simulink model "SHA256_simulink"  (R2015a)
settings: Solver=ode3  StartTime=0.0  StopTime=0  RelTol=1e-3
libraries: simulink x34, hdlsllib x24
settings Model: Creator=Hp  LastModifiedBy=Hp

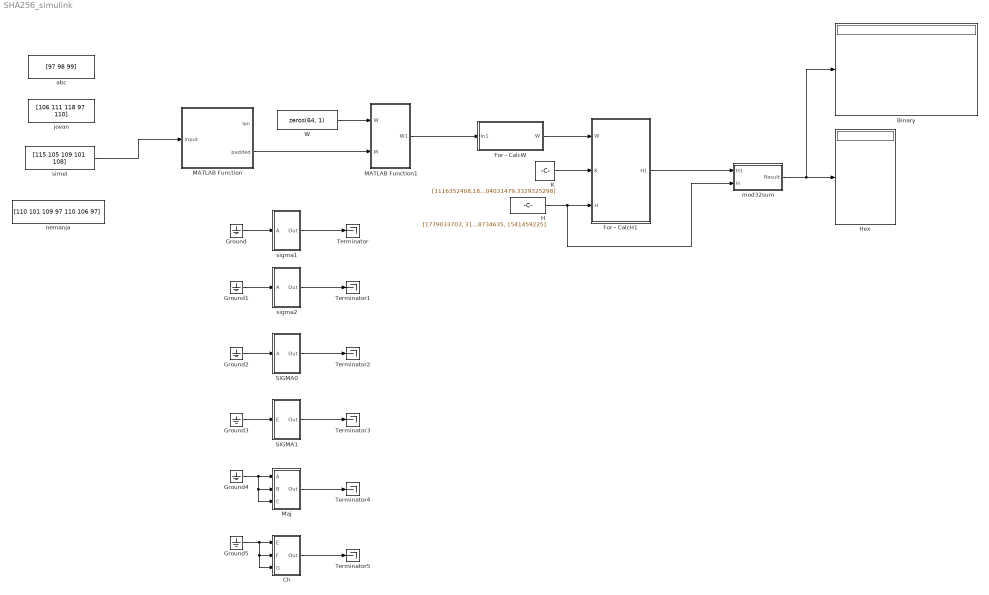
== system SHA256_simulink ==
  Binary : Display
      settings: Format=binary (Stored Integer)
  Ch : Subsystem
  For - CalcH1 : Subsystem  TreatAsAtomicUnit=on
  For - CalcW : Subsystem  TreatAsAtomicUnit=on
  Ground{,1..5} (6 alike) : Ground
  H : Constant  Value=[1779033703, 3144134277, 1013904242, 2773480762, 1359893119, 2600822924, 528734635, 1541459225]  OutDataTypeStr=uint32
  Hex : Display
      settings: Format=hex (Stored Integer)
  K : Constant  Value=[1116352408,1899447441,3049323471,3921009573,961987163,1508970993,2453635748,2870763221,3624381080,310598401,607225278,1426881987,1925078388,2162078206,2614888103,3248222580,3835390401,4022224774,264347078,604807628,770255983,1249150122,1555081692,1996064986,2554220882,2821834349,2952996808,3210313671,3336571891,3584528711,113926993,338241895,666307205,773529912,1294757372,1396182291,1695183700,1986661051,2177026350,2456956037,2730485921,2820302411,3259730800,3345764771,3516065817,3600352804,4094571909,275423344,430227734,506948616,659060556,883997877,958139571,1322822218,1537002063,1747873779,1955562222,2024104815,2227730452,2361852424,2428436474,2756734187,3204031479,3329325298]  OutDataTypeStr=uint32
  MATLAB Function : MATLAB Function  TreatAsAtomicUnit=on
  MATLAB Function1 : MATLAB Function  TreatAsAtomicUnit=on
  Maj : Subsystem
  SIGMA0 : Subsystem
  SIGMA1 : Subsystem
  Terminator{,1..5} (6 alike) : Terminator
  W : Constant  Value=zeros(64, 1)  VectorParams1D=off  OutDataTypeStr=uint32
  abc : Constant  Value=[97 98 99]
  jovan : Constant  Value=[106 111 118 97 110]
  mod32sum : Subsystem
  nemanja : Constant  Value=[110 101 109 97 110 106 97]
  "sigma1 " : Subsystem
  sigma2 : Subsystem
  "simel " : Constant  Value=[115 105 109 101 108]
  wires:
  W/1 -> MATLAB Function1/1(W)
  MATLAB Function/2(padded) -> MATLAB Function1/2(M)
  For - CalcW/1(W) -> For - CalcH1/1(W)
  K/1 -> For - CalcH1/2(K)
  For - CalcH1/1(H1) -> mod32sum/1(H1)
  mod32sum/1(Result) -> Binary/1, Hex/1
  H/1 -> mod32sum/2(H), For - CalcH1/3(H)
  Ground/1 -> "sigma1 "/1(A)
  Ground1/1 -> sigma2/1(A)
  Ground2/1 -> SIGMA0/1(A)
  Ground3/1 -> SIGMA1/1(E)
  Ground4/1 -> Maj/3(C), Maj/2(B), Maj/1(A)
  Ground5/1 -> Ch/3(G), Ch/2(F), Ch/1(E)
  "sigma1 "/1(Out) -> Terminator/1
  sigma2/1(Out) -> Terminator1/1
  SIGMA0/1(Out) -> Terminator2/1
  SIGMA1/1(Out) -> Terminator3/1
  Maj/1(Out) -> Terminator4/1
  Ch/1(Out) -> Terminator5/1
  "simel "/1 -> MATLAB Function/1(input)
  MATLAB Function1/1(W1) -> For - CalcW/1(In1)

== system SHA256_simulink/Ch ==
  E : Inport  OutDataTypeStr=uint32
  F : Inport  Port=2  OutDataTypeStr=uint32
  G : Inport  Port=3  OutDataTypeStr=uint32
  Bitwise Operator1 : simulink/Logic and Bit Operations/Bitwise Operator  logicop=AND  UseBitMask=off  NumInputPorts=2  BitMask=bin2dec('11011001')  BitMaskRealWorld=Stored Integer
  Bitwise Operator2 : simulink/Logic and Bit Operations/Bitwise Operator  logicop=NOT  UseBitMask=off  BitMask=bin2dec('11011001')  BitMaskRealWorld=Stored Integer
  Bitwise Operator3 : simulink/Logic and Bit Operations/Bitwise Operator  logicop=AND  UseBitMask=off  NumInputPorts=2  BitMask=bin2dec('11011001')  BitMaskRealWorld=Stored Integer
  Bitwise Operator5 : simulink/Logic and Bit Operations/Bitwise Operator  logicop=XOR  UseBitMask=off  NumInputPorts=2  BitMask=bin2dec('11011001')  BitMaskRealWorld=Stored Integer
  Out : Outport  OutDataTypeStr=uint32
  wires:
  E/1 -> Bitwise Operator2/1, Bitwise Operator1/1
  F/1 -> Bitwise Operator1/2
  Bitwise Operator5/1 -> Out/1
  G/1 -> Bitwise Operator3/2
  Bitwise Operator2/1 -> Bitwise Operator3/1
  Bitwise Operator3/1 -> Bitwise Operator5/2
  Bitwise Operator1/1 -> Bitwise Operator5/1

== system SHA256_simulink/For - CalcH1 ==
  W : Inport
  K : Inport  Port=2
  H : Inport  Port=3
  Calc H1 : Subsystem
  For Iterator : ForIterator  IterationLimit=64
  Selector : Selector  InputPortWidth=64  IndexOptions=Index vector (port)  Indices=[1 3]
  Selector1 : Selector  InputPortWidth=64  IndexOptions=Index vector (port)  Indices=[1 3]
  H1 : Outport
  wires:
  K/1 -> Selector/1
  W/1 -> Selector1/1
  For Iterator/1 -> Selector/2, Selector1/2
  Selector/1 -> Calc H1/2(Ki)
  Selector1/1 -> Calc H1/3(Wi)
  H/1 -> Calc H1/1(H)
  Calc H1/1(H1) -> H1/1

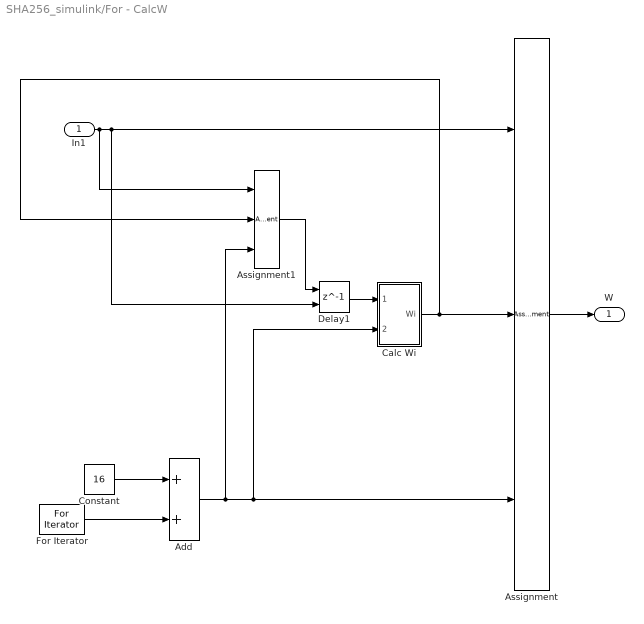
== system SHA256_simulink/For - CalcW ==
  In1 : Inport
  Add : Sum
  Assignment : Assignment  DiagnosticForDimensions=Warning  IndexOptions=Index vector (port)
  Assignment1 : Assignment  DiagnosticForDimensions=Warning  IndexOptions=Index vector (port)
  Calc Wi : Subsystem
  Constant : Constant  Value=16
  Delay1 : Delay  DelayLength=1  InitialConditionSource=Input port  InitialCondition=0
      settings: InputPortMap=u0,p4
  For Iterator : ForIterator  IterationLimit=48
  W : Outport
  wires:
  In1/1 -> Delay1/2, Assignment/1, Assignment1/1
  Add/1 -> Assignment1/3, Calc Wi/2(Index), Assignment/3
  Constant/1 -> Add/1
  For Iterator/1 -> Add/2
  Calc Wi/1(Wi) -> Assignment1/2, Assignment/2
  Delay1/1 -> Calc Wi/1(Array)
  Assignment1/1 -> Delay1/1
  Assignment/1 -> W/1

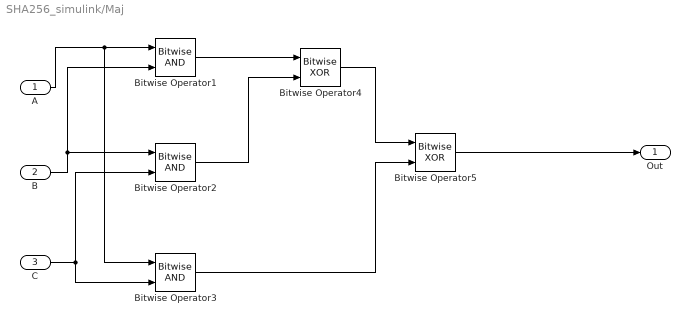
== system SHA256_simulink/Maj ==
  A : Inport  OutDataTypeStr=uint32
  B : Inport  Port=2  OutDataTypeStr=uint32
  C : Inport  Port=3  OutDataTypeStr=uint32
  Bitwise Operator1 : simulink/Logic and Bit Operations/Bitwise Operator  logicop=AND  UseBitMask=off  NumInputPorts=2  BitMask=bin2dec('11011001')  BitMaskRealWorld=Stored Integer
  Bitwise Operator2 : simulink/Logic and Bit Operations/Bitwise Operator  logicop=AND  UseBitMask=off  NumInputPorts=2  BitMask=bin2dec('11011001')  BitMaskRealWorld=Stored Integer
  Bitwise Operator3 : simulink/Logic and Bit Operations/Bitwise Operator  logicop=AND  UseBitMask=off  NumInputPorts=2  BitMask=bin2dec('11011001')  BitMaskRealWorld=Stored Integer
  Bitwise Operator4 : simulink/Logic and Bit Operations/Bitwise Operator  logicop=XOR  UseBitMask=off  NumInputPorts=2  BitMask=bin2dec('11011001')  BitMaskRealWorld=Stored Integer
  Bitwise Operator5 : simulink/Logic and Bit Operations/Bitwise Operator  logicop=XOR  UseBitMask=off  NumInputPorts=2  BitMask=bin2dec('11011001')  BitMaskRealWorld=Stored Integer
  Out : Outport  OutDataTypeStr=uint32
  wires:
  A/1 -> Bitwise Operator1/1, Bitwise Operator3/1
  B/1 -> Bitwise Operator2/1, Bitwise Operator1/2
  C/1 -> Bitwise Operator2/2, Bitwise Operator3/2
  Bitwise Operator1/1 -> Bitwise Operator4/1
  Bitwise Operator2/1 -> Bitwise Operator4/2
  Bitwise Operator3/1 -> Bitwise Operator5/2
  Bitwise Operator4/1 -> Bitwise Operator5/1
  Bitwise Operator5/1 -> Out/1

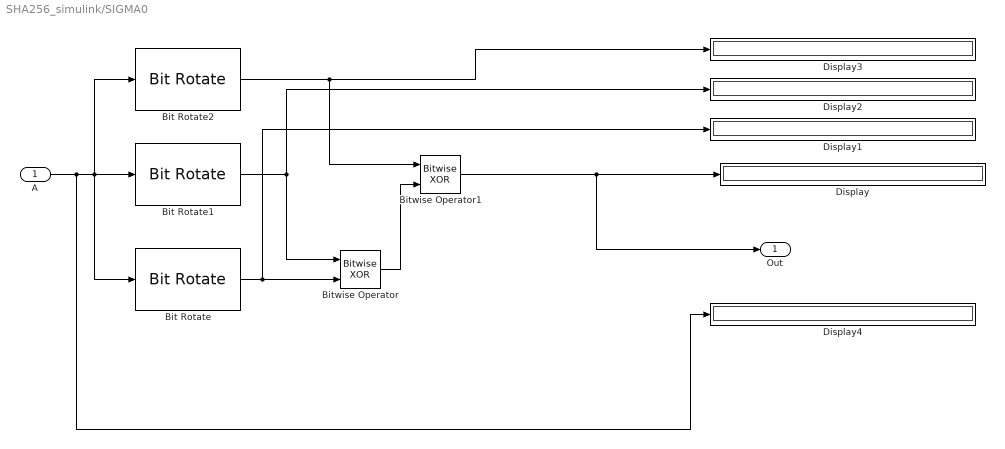
== system SHA256_simulink/SIGMA0 ==
  A : Inport  OutDataTypeStr=uint32
  Bit Rotate : hdlsllib/HDL Operations/Bit Rotate  mode=Rotate Right  N=22
  Bit Rotate1 : hdlsllib/HDL Operations/Bit Rotate  mode=Rotate Right  N=13
  Bit Rotate2 : hdlsllib/HDL Operations/Bit Rotate  mode=Rotate Right  N=2
  Bitwise Operator : simulink/Logic and Bit Operations/Bitwise Operator  logicop=XOR  UseBitMask=off  NumInputPorts=2  BitMask=bin2dec('11011001')  BitMaskRealWorld=Stored Integer
  Bitwise Operator1 : simulink/Logic and Bit Operations/Bitwise Operator  logicop=XOR  UseBitMask=off  NumInputPorts=2  BitMask=bin2dec('11011001')  BitMaskRealWorld=Stored Integer
  Display{,1..4} (5 alike) : Display
      Display settings: Format=hex (Stored Integer)
      Display1 settings: Format=binary (Stored Integer)
      Display2 settings: Format=binary (Stored Integer)
      Display3 settings: Format=binary (Stored Integer)
      Display4 settings: Format=binary (Stored Integer)
  Out : Outport  OutDataTypeStr=uint32
  wires:
  Bitwise Operator1/1 -> Out/1, Display/1
  Bitwise Operator/1 -> Bitwise Operator1/2
  A/1 -> Display4/1, Bit Rotate1/1, Bit Rotate2/1, Bit Rotate/1
  Bit Rotate/1 -> Display1/1, Bitwise Operator/2
  Bit Rotate2/1 -> Bitwise Operator1/1, Display3/1
  Bit Rotate1/1 -> Display2/1, Bitwise Operator/1

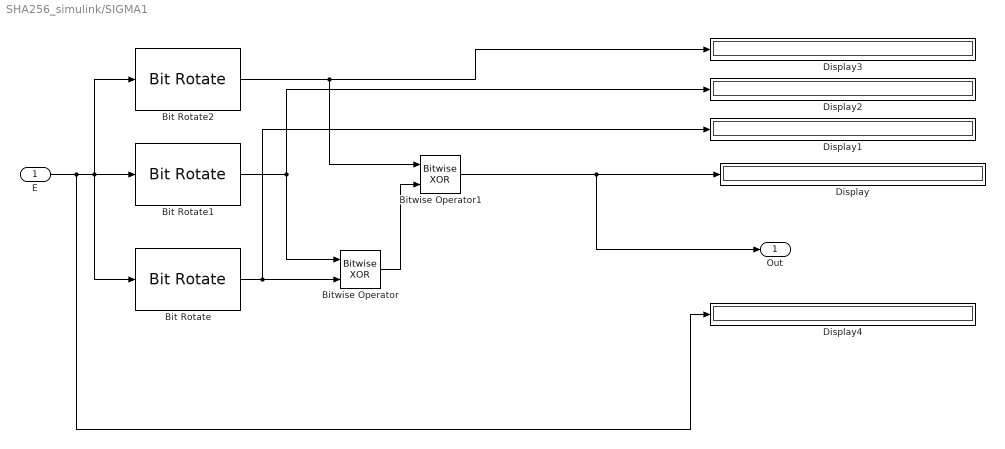
== system SHA256_simulink/SIGMA1 ==
  E : Inport  OutDataTypeStr=uint32
  Bit Rotate : hdlsllib/HDL Operations/Bit Rotate  mode=Rotate Right  N=25
  Bit Rotate1 : hdlsllib/HDL Operations/Bit Rotate  mode=Rotate Right  N=11
  Bit Rotate2 : hdlsllib/HDL Operations/Bit Rotate  mode=Rotate Right  N=6
  Bitwise Operator : simulink/Logic and Bit Operations/Bitwise Operator  logicop=XOR  UseBitMask=off  NumInputPorts=2  BitMask=bin2dec('11011001')  BitMaskRealWorld=Stored Integer
  Bitwise Operator1 : simulink/Logic and Bit Operations/Bitwise Operator  logicop=XOR  UseBitMask=off  NumInputPorts=2  BitMask=bin2dec('11011001')  BitMaskRealWorld=Stored Integer
  Display{,1..4} (5 alike) : Display
      Display settings: Format=hex (Stored Integer)
      Display1 settings: Format=binary (Stored Integer)
      Display2 settings: Format=binary (Stored Integer)
      Display3 settings: Format=binary (Stored Integer)
      Display4 settings: Format=binary (Stored Integer)
  Out : Outport  OutDataTypeStr=uint32
  wires:
  Bitwise Operator1/1 -> Out/1, Display/1
  Bitwise Operator/1 -> Bitwise Operator1/2
  E/1 -> Display4/1, Bit Rotate1/1, Bit Rotate2/1, Bit Rotate/1
  Bit Rotate/1 -> Display1/1, Bitwise Operator/2
  Bit Rotate2/1 -> Bitwise Operator1/1, Display3/1
  Bit Rotate1/1 -> Display2/1, Bitwise Operator/1

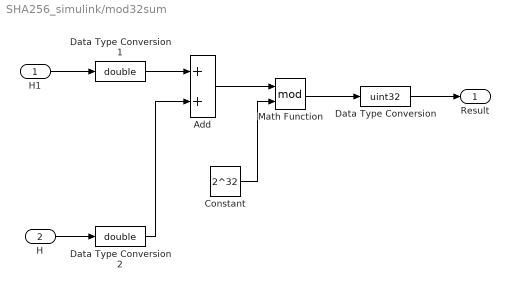
== system SHA256_simulink/mod32sum ==
  H1 : Inport
  H : Inport  Port=2
  Add : Sum
  Constant : Constant  Value=2^32
  Data Type Conversion : DataTypeConversion  OutDataTypeStr=uint32
  Data Type Conversion1 : DataTypeConversion  OutDataTypeStr=double
  Data Type Conversion2 : DataTypeConversion  OutDataTypeStr=double
  Math Function : Math  Operator=mod  SaturateOnIntegerOverflow=on
  Result : Outport
  wires:
  H1/1 -> Data Type Conversion1/1
  H/1 -> Data Type Conversion2/1
  Math Function/1 -> Data Type Conversion/1
  Add/1 -> Math Function/1
  Constant/1 -> Math Function/2
  Data Type Conversion/1 -> Result/1
  Data Type Conversion1/1 -> Add/1
  Data Type Conversion2/1 -> Add/2

== system SHA256_simulink/sigma1  ==
  A : Inport  OutDataTypeStr=uint32
  Bit Rotate1 : hdlsllib/HDL Operations/Bit Rotate  mode=Rotate Right  N=18
  Bit Rotate2 : hdlsllib/HDL Operations/Bit Rotate  mode=Rotate Right  N=7
  Bit Shift : hdlsllib/HDL Operations/Bit Shift  mode=Shift Right Logical  N=3
  Bitwise Operator : simulink/Logic and Bit Operations/Bitwise Operator  logicop=XOR  UseBitMask=off  NumInputPorts=2  BitMask=bin2dec('11011001')  BitMaskRealWorld=Stored Integer
  Bitwise Operator1 : simulink/Logic and Bit Operations/Bitwise Operator  logicop=XOR  UseBitMask=off  NumInputPorts=2  BitMask=bin2dec('11011001')  BitMaskRealWorld=Stored Integer
  Out : Outport  OutDataTypeStr=uint32
  wires:
  Bitwise Operator1/1 -> Out/1
  Bitwise Operator/1 -> Bitwise Operator1/2
  A/1 -> Bit Shift/1, Bit Rotate1/1, Bit Rotate2/1
  Bit Shift/1 -> Bitwise Operator/2
  Bit Rotate2/1 -> Bitwise Operator1/1
  Bit Rotate1/1 -> Bitwise Operator/1

== system SHA256_simulink/sigma2 ==
  A : Inport  OutDataTypeStr=uint32
  Bit Rotate1 : hdlsllib/HDL Operations/Bit Rotate  mode=Rotate Right  N=19
  Bit Rotate2 : hdlsllib/HDL Operations/Bit Rotate  mode=Rotate Right  N=17
  Bit Shift : hdlsllib/HDL Operations/Bit Shift  mode=Shift Right Logical  N=10
  Bitwise Operator : simulink/Logic and Bit Operations/Bitwise Operator  logicop=XOR  UseBitMask=off  NumInputPorts=2  BitMask=bin2dec('11011001')  BitMaskRealWorld=Stored Integer
  Bitwise Operator1 : simulink/Logic and Bit Operations/Bitwise Operator  logicop=XOR  UseBitMask=off  NumInputPorts=2  BitMask=bin2dec('11011001')  BitMaskRealWorld=Stored Integer
  Out : Outport  OutDataTypeStr=uint32
  wires:
  Bitwise Operator/1 -> Bitwise Operator1/2
  A/1 -> Bit Shift/1, Bit Rotate1/1, Bit Rotate2/1
  Bit Shift/1 -> Bitwise Operator/2
  Bit Rotate2/1 -> Bitwise Operator1/1
  Bit Rotate1/1 -> Bitwise Operator/1
  Bitwise Operator1/1 -> Out/1

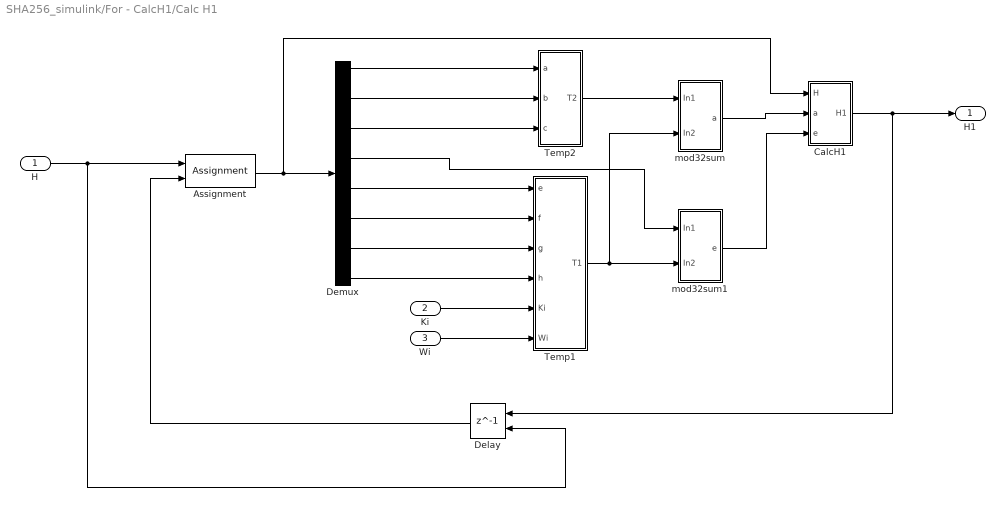
== system SHA256_simulink/For - CalcH1/Calc H1 ==
  H : Inport
  Ki : Inport  Port=2
  Wi : Inport  Port=3
  Assignment : Assignment  DiagnosticForDimensions=Warning  IndexOptions=Assign all
  CalcH1 : Subsystem
  Delay : Delay  DelayLength=1  InitialConditionSource=Input port  InitialCondition=0
      settings: InputPortMap=u0,p4
  Demux : Demux  Outputs=8
  Temp1 : Subsystem
  Temp2 : Subsystem
  mod32sum : Subsystem
  mod32sum1 : Subsystem
  H1 : Outport
  wires:
  Demux/5 -> Temp1/1(e)
  Demux/6 -> Temp1/2(f)
  Demux/7 -> Temp1/3(g)
  Demux/8 -> Temp1/4(h)
  Ki/1 -> Temp1/5(Ki)
  Wi/1 -> Temp1/6(Wi)
  Demux/1 -> Temp2/1(a)
  Demux/2 -> Temp2/2(b)
  Demux/3 -> Temp2/3(c)
  Temp2/1(T2) -> mod32sum/1(In1)
  Temp1/1(T1) -> mod32sum/2(In2), mod32sum1/2(In2)
  Demux/4 -> mod32sum1/1(In1)
  mod32sum1/1(e) -> CalcH1/3(e)
  H/1 -> Delay/2, Assignment/1
  Assignment/1 -> CalcH1/1(H), Demux/1
  CalcH1/1(H1) -> Delay/1, H1/1
  Delay/1 -> Assignment/2
  mod32sum/1(a) -> CalcH1/2(a)

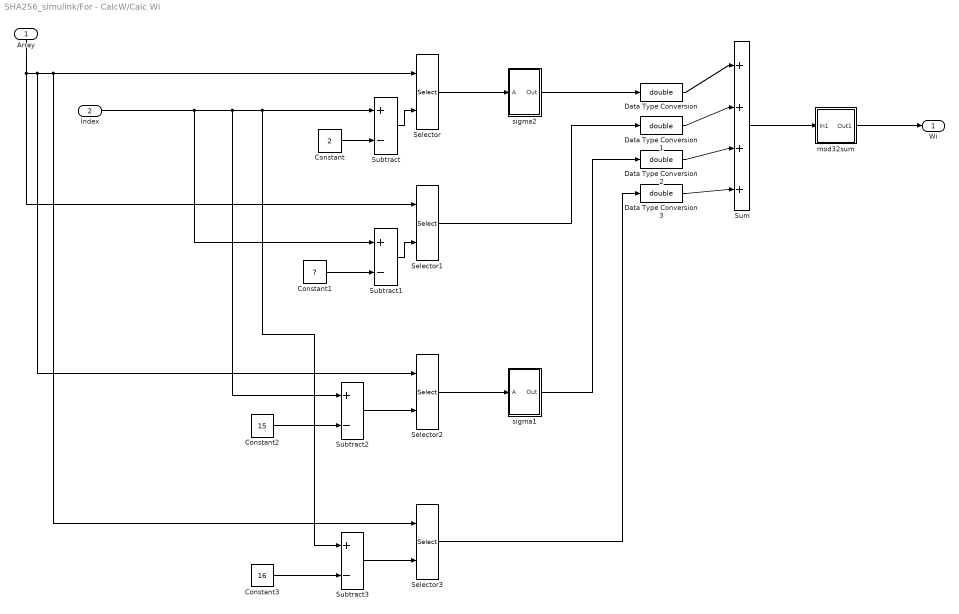
== system SHA256_simulink/For - CalcW/Calc Wi ==
  Array : Inport
  Index : Inport  Port=2
  Constant : Constant  Value=2  OutDataTypeStr=uint32
  Constant1 : Constant  Value=7  OutDataTypeStr=uint32
  Constant2 : Constant  Value=15  OutDataTypeStr=uint32
  Constant3 : Constant  Value=16  OutDataTypeStr=uint32
  Data Type Conversion{,1..3} (4 alike) : DataTypeConversion  OutDataTypeStr=double
  Selector{,1..3} (4 alike) : Selector  InputPortWidth=64  IndexOptions=Index vector (port)  Indices=[1 3]
  Subtract{,1..3} (4 alike) : Sum  Inputs=+-  OutDataTypeStr=uint32
  Sum : Sum  Inputs=|++++
  mod32sum : Subsystem
  "sigma1 " : Subsystem
  sigma2 : Subsystem
  Wi : Outport
  wires:
  Constant/1 -> Subtract/2
  Subtract/1 -> Selector/2
  Subtract1/1 -> Selector1/2
  Constant1/1 -> Subtract1/2
  Subtract2/1 -> Selector2/2
  Constant2/1 -> Subtract2/2
  Array/1 -> Selector2/1, Selector3/1, Selector/1, Selector1/1
  Index/1 -> Subtract2/1, Subtract3/1, Subtract/1, Subtract1/1
  Subtract3/1 -> Selector3/2
  Constant3/1 -> Subtract3/2
  Selector/1 -> sigma2/1(A)
  Selector2/1 -> "sigma1 "/1(A)
  Sum/1 -> mod32sum/1(In1)
  sigma2/1(Out) -> Data Type Conversion/1
  Selector1/1 -> Data Type Conversion1/1
  "sigma1 "/1(Out) -> Data Type Conversion2/1
  Selector3/1 -> Data Type Conversion3/1
  mod32sum/1(Out1) -> Wi/1
  Data Type Conversion/1 -> Sum/1
  Data Type Conversion1/1 -> Sum/2
  Data Type Conversion2/1 -> Sum/3
  Data Type Conversion3/1 -> Sum/4

== system SHA256_simulink/For - CalcH1/Calc H1/CalcH1 ==
  H : Inport
  a : Inport  Port=2
  e : Inport  Port=3
  Demux : Demux  Outputs=8
  To Workspace : ToWorkspace  VariableName=simout  SaveFormat=Timeseries  SampleTime=-1
  Vector Concatenate : Concatenate  NumInputs=8
  H1 : Outport
  wires:
  H/1 -> Demux/1
  Demux/1 -> Vector Concatenate/2
  a/1 -> Vector Concatenate/1
  Demux/2 -> Vector Concatenate/3
  Demux/3 -> Vector Concatenate/4
  e/1 -> Vector Concatenate/5
  Demux/5 -> Vector Concatenate/6
  Demux/6 -> Vector Concatenate/7
  Demux/7 -> Vector Concatenate/8
  Vector Concatenate/1 -> To Workspace/1, H1/1

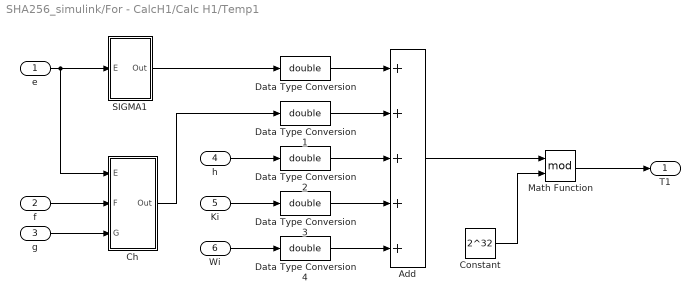
== system SHA256_simulink/For - CalcH1/Calc H1/Temp1 ==
  e : Inport
  f : Inport  Port=2
  g : Inport  Port=3
  h : Inport  Port=4
  Ki : Inport  Port=5
  Wi : Inport  Port=6
  Add : Sum  Inputs=+++++
  Ch : Subsystem
  Constant : Constant  Value=2^32
  Data Type Conversion{,1..4} (5 alike) : DataTypeConversion  OutDataTypeStr=double
  Math Function : Math  Operator=mod  SaturateOnIntegerOverflow=on
  SIGMA1 : Subsystem
  T1 : Outport
  wires:
  f/1 -> Ch/2(F)
  g/1 -> Ch/3(G)
  e/1 -> SIGMA1/1(E), Ch/1(E)
  SIGMA1/1(Out) -> Data Type Conversion/1
  Ch/1(Out) -> Data Type Conversion1/1
  h/1 -> Data Type Conversion2/1
  Ki/1 -> Data Type Conversion3/1
  Wi/1 -> Data Type Conversion4/1
  Data Type Conversion/1 -> Add/1
  Data Type Conversion1/1 -> Add/2
  Data Type Conversion2/1 -> Add/3
  Data Type Conversion3/1 -> Add/4
  Data Type Conversion4/1 -> Add/5
  Add/1 -> Math Function/1
  Constant/1 -> Math Function/2
  Math Function/1 -> T1/1

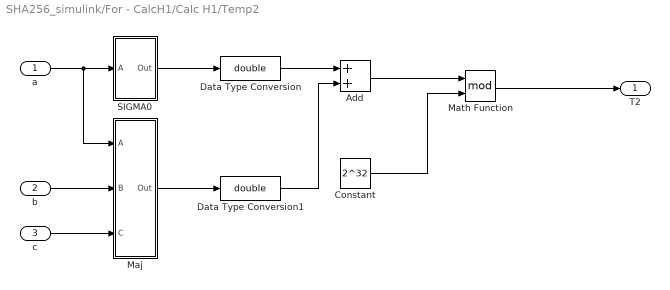
== system SHA256_simulink/For - CalcH1/Calc H1/Temp2 ==
  a : Inport
  b : Inport  Port=2
  c : Inport  Port=3
  Add : Sum
  Constant : Constant  Value=2^32
  Data Type Conversion : DataTypeConversion  OutDataTypeStr=double
  Data Type Conversion1 : DataTypeConversion  OutDataTypeStr=double
  Maj : Subsystem
  Math Function : Math  Operator=mod  SaturateOnIntegerOverflow=on
  SIGMA0 : Subsystem
  T2 : Outport
  wires:
  b/1 -> Maj/2(B)
  c/1 -> Maj/3(C)
  a/1 -> SIGMA0/1(A), Maj/1(A)
  Maj/1(Out) -> Data Type Conversion1/1
  SIGMA0/1(Out) -> Data Type Conversion/1
  Data Type Conversion/1 -> Add/1
  Data Type Conversion1/1 -> Add/2
  Add/1 -> Math Function/1
  Constant/1 -> Math Function/2
  Math Function/1 -> T2/1

== system SHA256_simulink/For - CalcH1/Calc H1/mod32sum ==
  In1 : Inport
  In2 : Inport  Port=2
  Add : Sum
  Constant : Constant  Value=2^32
  Data Type Conversion : DataTypeConversion  OutDataTypeStr=uint32
  Math Function : Math  Operator=mod  SaturateOnIntegerOverflow=on
  a : Outport
  wires:
  In1/1 -> Add/1
  In2/1 -> Add/2
  Math Function/1 -> Data Type Conversion/1
  Add/1 -> Math Function/1
  Constant/1 -> Math Function/2
  Data Type Conversion/1 -> a/1

== system SHA256_simulink/For - CalcH1/Calc H1/mod32sum1 ==
  In1 : Inport
  In2 : Inport  Port=2
  Add : Sum
  Constant : Constant  Value=2^32
  Data Type Conversion : DataTypeConversion  OutDataTypeStr=uint32
  Math Function : Math  Operator=mod  SaturateOnIntegerOverflow=on
  e : Outport
  wires:
  In1/1 -> Add/1
  In2/1 -> Add/2
  Math Function/1 -> Data Type Conversion/1
  Add/1 -> Math Function/1
  Constant/1 -> Math Function/2
  Data Type Conversion/1 -> e/1

== system SHA256_simulink/For - CalcW/Calc Wi/mod32sum ==
  In1 : Inport
  Constant : Constant  Value=2^32
  Data Type Conversion : DataTypeConversion  OutDataTypeStr=uint32
  Math Function : Math  Operator=mod  SaturateOnIntegerOverflow=on
  Out1 : Outport
  wires:
  Math Function/1 -> Data Type Conversion/1
  Constant/1 -> Math Function/2
  Data Type Conversion/1 -> Out1/1
  In1/1 -> Math Function/1

== system SHA256_simulink/For - CalcW/Calc Wi/sigma1  ==
  A : Inport  OutDataTypeStr=uint32
  Bit Rotate1 : hdlsllib/HDL Operations/Bit Rotate  mode=Rotate Right  N=18
  Bit Rotate2 : hdlsllib/HDL Operations/Bit Rotate  mode=Rotate Right  N=7
  Bit Shift : hdlsllib/HDL Operations/Bit Shift  mode=Shift Right Logical  N=3
  Bitwise Operator : simulink/Logic and Bit Operations/Bitwise Operator  logicop=XOR  UseBitMask=off  NumInputPorts=2  BitMask=bin2dec('11011001')  BitMaskRealWorld=Stored Integer
  Bitwise Operator1 : simulink/Logic and Bit Operations/Bitwise Operator  logicop=XOR  UseBitMask=off  NumInputPorts=2  BitMask=bin2dec('11011001')  BitMaskRealWorld=Stored Integer
  Out : Outport  OutDataTypeStr=uint32
  wires:
  Bitwise Operator1/1 -> Out/1
  Bitwise Operator/1 -> Bitwise Operator1/2
  A/1 -> Bit Shift/1, Bit Rotate1/1, Bit Rotate2/1
  Bit Shift/1 -> Bitwise Operator/2
  Bit Rotate2/1 -> Bitwise Operator1/1
  Bit Rotate1/1 -> Bitwise Operator/1

== system SHA256_simulink/For - CalcW/Calc Wi/sigma2 ==
  A : Inport  OutDataTypeStr=uint32
  Bit Rotate1 : hdlsllib/HDL Operations/Bit Rotate  mode=Rotate Right  N=19
  Bit Rotate2 : hdlsllib/HDL Operations/Bit Rotate  mode=Rotate Right  N=17
  Bit Shift : hdlsllib/HDL Operations/Bit Shift  mode=Shift Right Logical  N=10
  Bitwise Operator : simulink/Logic and Bit Operations/Bitwise Operator  logicop=XOR  UseBitMask=off  NumInputPorts=2  BitMask=bin2dec('11011001')  BitMaskRealWorld=Stored Integer
  Bitwise Operator1 : simulink/Logic and Bit Operations/Bitwise Operator  logicop=XOR  UseBitMask=off  NumInputPorts=2  BitMask=bin2dec('11011001')  BitMaskRealWorld=Stored Integer
  Out : Outport  OutDataTypeStr=uint32
  wires:
  Bitwise Operator/1 -> Bitwise Operator1/2
  A/1 -> Bit Shift/1, Bit Rotate1/1, Bit Rotate2/1
  Bit Shift/1 -> Bitwise Operator/2
  Bit Rotate2/1 -> Bitwise Operator1/1
  Bit Rotate1/1 -> Bitwise Operator/1
  Bitwise Operator1/1 -> Out/1

== system SHA256_simulink/For - CalcH1/Calc H1/Temp1/Ch ==
  E : Inport  OutDataTypeStr=uint32
  F : Inport  Port=2  OutDataTypeStr=uint32
  G : Inport  Port=3  OutDataTypeStr=uint32
  Bitwise Operator1 : simulink/Logic and Bit Operations/Bitwise Operator  logicop=AND  UseBitMask=off  NumInputPorts=2  BitMask=bin2dec('11011001')  BitMaskRealWorld=Stored Integer
  Bitwise Operator2 : simulink/Logic and Bit Operations/Bitwise Operator  logicop=NOT  UseBitMask=off  BitMask=bin2dec('11011001')  BitMaskRealWorld=Stored Integer
  Bitwise Operator3 : simulink/Logic and Bit Operations/Bitwise Operator  logicop=AND  UseBitMask=off  NumInputPorts=2  BitMask=bin2dec('11011001')  BitMaskRealWorld=Stored Integer
  Bitwise Operator5 : simulink/Logic and Bit Operations/Bitwise Operator  logicop=XOR  UseBitMask=off  NumInputPorts=2  BitMask=bin2dec('11011001')  BitMaskRealWorld=Stored Integer
  Out : Outport  OutDataTypeStr=uint32
  wires:
  E/1 -> Bitwise Operator2/1, Bitwise Operator1/1
  F/1 -> Bitwise Operator1/2
  Bitwise Operator5/1 -> Out/1
  G/1 -> Bitwise Operator3/2
  Bitwise Operator2/1 -> Bitwise Operator3/1
  Bitwise Operator3/1 -> Bitwise Operator5/2
  Bitwise Operator1/1 -> Bitwise Operator5/1

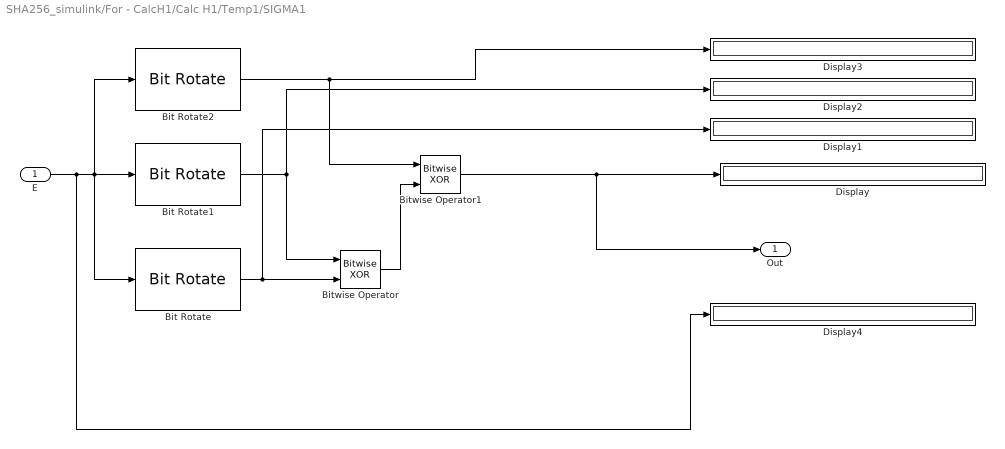
== system SHA256_simulink/For - CalcH1/Calc H1/Temp1/SIGMA1 ==
  E : Inport  OutDataTypeStr=uint32
  Bit Rotate : hdlsllib/HDL Operations/Bit Rotate  mode=Rotate Right  N=25
  Bit Rotate1 : hdlsllib/HDL Operations/Bit Rotate  mode=Rotate Right  N=11
  Bit Rotate2 : hdlsllib/HDL Operations/Bit Rotate  mode=Rotate Right  N=6
  Bitwise Operator : simulink/Logic and Bit Operations/Bitwise Operator  logicop=XOR  UseBitMask=off  NumInputPorts=2  BitMask=bin2dec('11011001')  BitMaskRealWorld=Stored Integer
  Bitwise Operator1 : simulink/Logic and Bit Operations/Bitwise Operator  logicop=XOR  UseBitMask=off  NumInputPorts=2  BitMask=bin2dec('11011001')  BitMaskRealWorld=Stored Integer
  Display{,1..4} (5 alike) : Display
      Display settings: Format=hex (Stored Integer)
      Display1 settings: Format=binary (Stored Integer)
      Display2 settings: Format=binary (Stored Integer)
      Display3 settings: Format=binary (Stored Integer)
      Display4 settings: Format=binary (Stored Integer)
  Out : Outport  OutDataTypeStr=uint32
  wires:
  Bitwise Operator1/1 -> Out/1, Display/1
  Bitwise Operator/1 -> Bitwise Operator1/2
  E/1 -> Display4/1, Bit Rotate1/1, Bit Rotate2/1, Bit Rotate/1
  Bit Rotate/1 -> Display1/1, Bitwise Operator/2
  Bit Rotate2/1 -> Bitwise Operator1/1, Display3/1
  Bit Rotate1/1 -> Display2/1, Bitwise Operator/1

== system SHA256_simulink/For - CalcH1/Calc H1/Temp2/Maj ==
  A : Inport  OutDataTypeStr=uint32
  B : Inport  Port=2  OutDataTypeStr=uint32
  C : Inport  Port=3  OutDataTypeStr=uint32
  Bitwise Operator1 : simulink/Logic and Bit Operations/Bitwise Operator  logicop=AND  UseBitMask=off  NumInputPorts=2  BitMask=bin2dec('11011001')  BitMaskRealWorld=Stored Integer
  Bitwise Operator2 : simulink/Logic and Bit Operations/Bitwise Operator  logicop=AND  UseBitMask=off  NumInputPorts=2  BitMask=bin2dec('11011001')  BitMaskRealWorld=Stored Integer
  Bitwise Operator3 : simulink/Logic and Bit Operations/Bitwise Operator  logicop=AND  UseBitMask=off  NumInputPorts=2  BitMask=bin2dec('11011001')  BitMaskRealWorld=Stored Integer
  Bitwise Operator4 : simulink/Logic and Bit Operations/Bitwise Operator  logicop=XOR  UseBitMask=off  NumInputPorts=2  BitMask=bin2dec('11011001')  BitMaskRealWorld=Stored Integer
  Bitwise Operator5 : simulink/Logic and Bit Operations/Bitwise Operator  logicop=XOR  UseBitMask=off  NumInputPorts=2  BitMask=bin2dec('11011001')  BitMaskRealWorld=Stored Integer
  Out : Outport  OutDataTypeStr=uint32
  wires:
  A/1 -> Bitwise Operator1/1, Bitwise Operator3/1
  B/1 -> Bitwise Operator2/1, Bitwise Operator1/2
  C/1 -> Bitwise Operator2/2, Bitwise Operator3/2
  Bitwise Operator1/1 -> Bitwise Operator4/1
  Bitwise Operator2/1 -> Bitwise Operator4/2
  Bitwise Operator3/1 -> Bitwise Operator5/2
  Bitwise Operator4/1 -> Bitwise Operator5/1
  Bitwise Operator5/1 -> Out/1

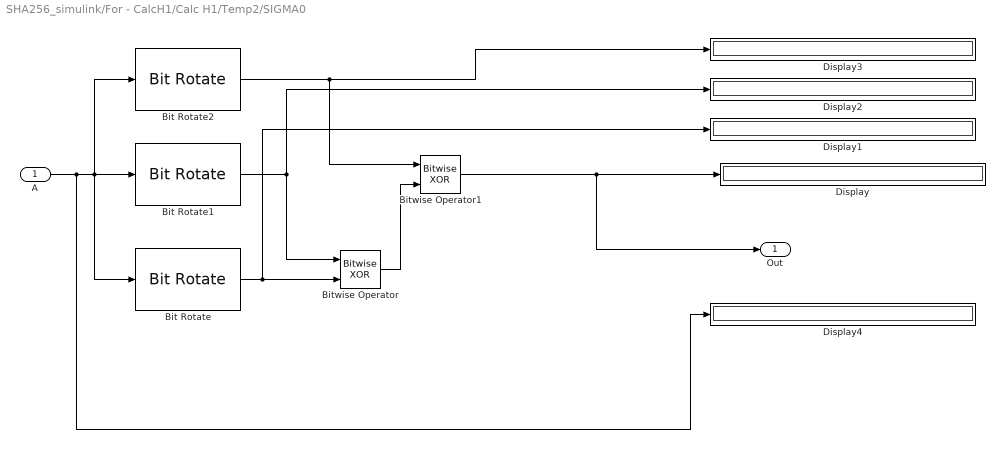
== system SHA256_simulink/For - CalcH1/Calc H1/Temp2/SIGMA0 ==
  A : Inport  OutDataTypeStr=uint32
  Bit Rotate : hdlsllib/HDL Operations/Bit Rotate  mode=Rotate Right  N=22
  Bit Rotate1 : hdlsllib/HDL Operations/Bit Rotate  mode=Rotate Right  N=13
  Bit Rotate2 : hdlsllib/HDL Operations/Bit Rotate  mode=Rotate Right  N=2
  Bitwise Operator : simulink/Logic and Bit Operations/Bitwise Operator  logicop=XOR  UseBitMask=off  NumInputPorts=2  BitMask=bin2dec('11011001')  BitMaskRealWorld=Stored Integer
  Bitwise Operator1 : simulink/Logic and Bit Operations/Bitwise Operator  logicop=XOR  UseBitMask=off  NumInputPorts=2  BitMask=bin2dec('11011001')  BitMaskRealWorld=Stored Integer
  Display{,1..4} (5 alike) : Display
      Display settings: Format=hex (Stored Integer)
      Display1 settings: Format=binary (Stored Integer)
      Display2 settings: Format=binary (Stored Integer)
      Display3 settings: Format=binary (Stored Integer)
      Display4 settings: Format=binary (Stored Integer)
  Out : Outport  OutDataTypeStr=uint32
  wires:
  Bitwise Operator1/1 -> Out/1, Display/1
  Bitwise Operator/1 -> Bitwise Operator1/2
  A/1 -> Display4/1, Bit Rotate1/1, Bit Rotate2/1, Bit Rotate/1
  Bit Rotate/1 -> Display1/1, Bitwise Operator/2
  Bit Rotate2/1 -> Bitwise Operator1/1, Display3/1
  Bit Rotate1/1 -> Display2/1, Bitwise Operator/1

== matlab function SHA256_simulink/MATLAB Function1 ==
  data: W input; W1 output; M input
function W1 = fcn(W, M)
    %#codegen
    W1 = uint32(zeros(1, 64));
    for j = 1:64
        % Prvih 16 redova rezervisano je za vrednosti u bloku M
        if(j > 0 && j <= 16)
            sum = uint32(zeros(1, 4));
            for i = 1:4
                sum(i) = M(1, 4 * (j - 1) + i);
            end
            conc = uint32(bitconcat(fi(sum, 0, 8, 0)));
            W1(j) = conc;       
        end
    end
end

== matlab function SHA256_simulink/MATLAB Function ==
  data: input input; len output; padded output
function [ len, padded ] = padding(input)
    %#codegen
    len = length(input);
    padded = uint32(zeros(1, 64));
    
    for i = 1:len
        padded(i) = input(i);
    end
    
    
    padded(len + 1) = 128;
    
    num = 1;
    
    while(num * 32 < len)
        padded(end - num + 1) = 255;
        num = num + 1;
    end
    
    padded(end - num + 1) = mod(len, 32) * 8;
    
    if(padded(end - num + 1) == 256)
        padded(end - num + 1) = 255;
    end
    
end
